simulink model "batu_boost120W_AKIM_KONTROL1"  (R2025a)
settings: Solver=ode23t  StartTime=0.0  StopTime=0.2  RelTol=1e-3
libraries: spsCurrentMeasurementLib x5, spsSeriesRLCBranchLib x3, spsMosfetLib x2, spsVoltageMeasurementLib x2, spsDCVoltageSourceLib x1, spsMeanLib x1, slpidlib x1, spsPWMGeneratorDCDCLib x1, sps_lib x1
settings Model: Creator=sagda  LastModifiedBy=sagda

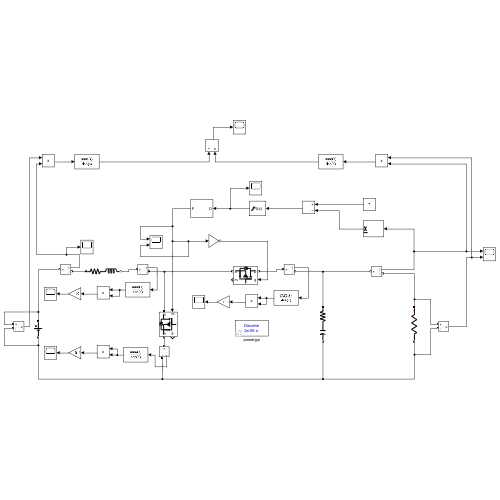
[thumbnail: Simulink's stored preview of the top-level diagram]
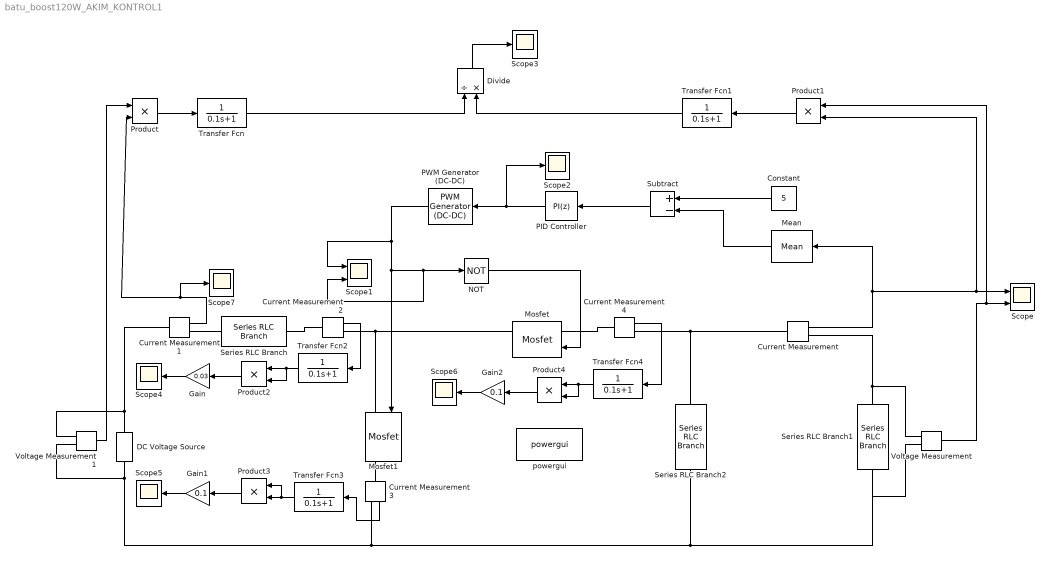
== system batu_boost120W_AKIM_KONTROL1 ==
  Constant : Constant  Value=5
  Current Measurement{,1..4} (5 alike) : spsCurrentMeasurementLib/Current Measurement  PhasorSimulation=off  OutputType=Complex  PSBequivalent=0
  DC Voltage Source : spsDCVoltageSourceLib/DC Voltage Source  Amplitude=24  Measurements=None
  Divide : Product  Inputs=/*
  Gain : Gain  Gain=0.03
  Gain1 : Gain  Gain=0.1
  Gain2 : Gain  Gain=0.1
  Mean : spsMeanLib/Mean  Freq=30000  Vinit=0  Ts=0
  Mosfet : spsMosfetLib/Mosfet  Ron=0.1  Lon=0  Rd=0.01  Vfd=0  IC=0  Rs=1e5  Cs=inf  Measurements=on
  Mosfet1 : spsMosfetLib/Mosfet  Ron=0.1  Lon=0  Rd=0.01  Vfd=0  IC=0  Rs=1e5  Cs=inf  Measurements=on
  NOT : Logic  Operator=NOT  IconShape=distinctive  AllPortsSameDT=off  OutDataTypeStr=boolean
  PID Controller : slpidlib/PID Controller  Controller=PI  Form=Parallel  TimeDomain=Discrete-time  UseExternalTs=off  SampleTime=2e-5  IntegratorMethod=Forward Euler  FilterMethod=Forward Euler  ControllerParametersSource=internal  P=0.001  I=5  UseKiTs=off  D=0  UseExternalDerivativeSource=off  N=100  UseFilter=on  TunerSelectOption=Transfer Function Based (PID Tuner App)  InitialConditionSource=internal  InitialConditionForIntegrator=0  InitialConditionForFilter=0  DifferentiatorICPrevScaledInput=0  ExternalReset=none  TrackingMode=off  Kt=1  LimitOutput=on  SatLimitsSource=internal  UpperSaturationLimit=0.9  LowerSaturationLimit=0  LinearizeAsGain=on  AntiWindupMode=clamping  Kb=1  LimitIntegrator=on  UpperIntegratorSaturationLimit=0.9  LowerIntegratorSaturationLimit=0  POutMin=[]  POutMax=[]  IOutMin=[]  IOutMax=[]  DOutMin=[]  DOutMax=[]  NOutMin=[]  NOutMax=[]  SumOutMin=[]  SumOutMax=[]  SaturationOutMin=[]  SaturationOutMax=[]  PParamMin=[]  PParamMax=[]  IParamMin=[]  IParamMax=[]  DParamMin=[]  DParamMax=[]  NParamMin=[]  NParamMax=[]  KbParamMin=[]  KbParamMax=[]  KtParamMin=[]  KtParamMax=[]  KbOutMin=[]  KbOutMax=[]  KtOutMin=[]  KtOutMax=[]  IntegratorOutMin=[]  IntegratorOutMax=[]  FilterOutMin=[]  FilterOutMax=[]  SumI1OutMin=[]  SumI1OutMax=[]  SumI2OutMin=[]  SumI2OutMax=[]  SumI3OutMin=[]  SumI3OutMax=[]  SumI4OutMin=[]  SumI4OutMax=[]  SumDOutMin=[]  SumDOutMax=[]  DifferentiatorOutMin=[]  DifferentiatorOutMax=[]  FilterDiffOutCoefMin=[]  FilterDiffOutCoefMax=[]  ReciprocalOutMin=[]  ReciprocalOutMax=[]  SumDenOutMin=[]  SumDenOutMax=[]  SumNumOutMin=[]  SumNumOutMax=[]  DivideOutMin=[]  DivideOutMax=[]  UdiffTsProdOutMin=[]  UdiffTsProdOutMax=[]  NTsProdOutMin=[]  NTsProdOutMax=[]  UintegralTsProdOutMin=[]  UintegralTsProdOutMax=[]  UngainTsProdOutMin=[]  UngainTsProdOutMax=[]  ClampingZeroOutDataTypeStr=Inherit: Inherit via back propagation  ClampingZeroOutMin=[]  ClampingZeroOutMax=[]  FilterDenConstantOutDataTypeStr=Inherit: Inherit via back propagation  FilterDenConstantOutMin=[]  FilterDenConstantOutMax=[]  PCopyOutDataTypeStr=Inherit: Inherit via back propagation  PCopyOutMin=[]  PCopyOutMax=[]  NCopyOutDataTypeStr=Inherit: Inherit via back propagation  NCopyOutMin=[]  NCopyOutMax=[]  IntegratorContinuousStateAttributes=''  IntegratorStateMustResolveToSignalObject=off  IntegratorRTWStateStorageClass=Auto  FilterContinuousStateAttributes=''  FilterStateMustResolveToSignalObject=off  FilterRTWStateStorageClass=Auto  ParallelPVariant=InternalParameters  IdealPVariant=Disabled  IVariant=InternalParameters  DVariant=Disabled  IntegratorVariant=Discrete  SatVariant=Enabled  AWVariant=DiscClampingParallel  PCopyVariant=Disabled  TRVariant=Disabled  FdbkBlocksVariant=Forward  IdealPFdbkVariant=Disabled  SatFdbkVariant=Disabled  DerivativeFilterVariant=Disabled  NVariant=Disabled  NCopyVariant=Disabled_SignalSpec  FilterICVariant=Disabled  IntegratorICVariant=InternalICs  ExternalResetVariant=Disabled  TRSumVariant=Passthrough  SumFdbkVariant=Disabled  SumVariant=Sum_PI  TsampFilterVariant=InternalTs  TsampNgainVariant=Passthrough  TsampIntegralVariant=Disabled_SignalSpec  ExternalSaturationOutDataTypeStr=Inherit: Same as second input  DerivativeSourceVariant=Disabled  PreIntVariant=InternalPreInt
  PWM Generator (DC-DC) : spsPWMGeneratorDCDCLib/PWM Generator (DC-DC)  Fsw=5000  Ts=0
  Product{,1..4} (5 alike) : Product
  Scope : Scope  NumInputPorts=2
      settings: ActiveDisplayYMinimum=-127.10682786797719  ActiveDisplayYMaximum=354.81313119342929
  Scope1 : Scope  NumInputPorts=2
      settings: ActiveDisplayYMinimum=0.054276  ActiveDisplayYMaximum=2.1879
  Scope{2..7} (6 alike) : Scope
      Scope2 settings: ActiveDisplayYMinimum=-0.12269  ActiveDisplayYMaximum=1.6409  DataLoggingVariableName=ScopeData2
      Scope3 settings: ActiveDisplayYMinimum=0.94291  ActiveDisplayYMaximum=0.95963  DataLoggingVariableName=ScopeData3
      Scope4 settings: ActiveDisplayYMinimum=0.78588  ActiveDisplayYMaximum=5.2873  DataLoggingVariableName=ScopeData4
      Scope5 settings: ActiveDisplayYMinimum=-0.94871  ActiveDisplayYMaximum=4.3636  DataLoggingVariableName=ScopeData5
      Scope6 settings: ActiveDisplayYMinimum=-13.0591  ActiveDisplayYMaximum=15.0829  DataLoggingVariableName=ScopeData6
      Scope7 settings: ActiveDisplayYMinimum=7.4423  ActiveDisplayYMaximum=25.7483  DataLoggingVariableName=ScopeData7
  Series RLC Branch : spsSeriesRLCBranchLib/Series RLC Branch  LConnTagsString=__new0  RConnTagsString=__new0  BranchType=RL  Resistance=0.03  Inductance=200e-6  SetiL0=off  InitialCurrent=0  Capacitance=1e-6  Setx0=off  InitialVoltage=0  Measurements=None
  Series RLC Branch1 : spsSeriesRLCBranchLib/Series RLC Branch  LConnTagsString=__new0  RConnTagsString=__new0  BranchType=R  Resistance=9.6  Inductance=1e-3  SetiL0=off  InitialCurrent=0  Capacitance=1e-6  Setx0=off  InitialVoltage=0  Measurements=None
  Series RLC Branch2 : spsSeriesRLCBranchLib/Series RLC Branch  LConnTagsString=__new0  RConnTagsString=__new0  BranchType=RC  Resistance=0.02  Inductance=1e-3  SetiL0=off  InitialCurrent=0  Capacitance=220e-6  Setx0=off  InitialVoltage=0  Measurements=None
  Subtract : Sum  Inputs=+-
  Transfer Fcn{,1..4} (5 alike) : TransferFcn  Denominator=[0.1 1]
  Voltage Measurement : spsVoltageMeasurementLib/Voltage Measurement  PhasorSimulation=off  OutputType=Complex  PSBequivalent=0
  Voltage Measurement1 : spsVoltageMeasurementLib/Voltage Measurement  PhasorSimulation=off  OutputType=Complex  PSBequivalent=0
  powergui : sps_lib/powergui  Priority=1  SimulationMode=Discrete  SampleTime=2e-6  frequency=60  Iterations=50  frequencyindice=0  Pbase=100e6  ErrMax=1e-4  UnitsV=kV  UnitsW=MW  buscounter=0  FunctionMessages=off  echomessages=off  EnableUseOfTLC=off  CurrentSourceSwitches=off  DisableSnubberDevices=off  DisableRonSwitches=off  DisableVfSwitches=off  DisplayEquations=off  AutomaticDiscreteSolvers=off  SolverType=Tustin/Backward Euler (TBE)  Interpol=off  ExternalGateDelay=off  methode=off  Ts=100  x0status=blocks  SPID=on  SwTol=0  HookPort=off  NonlinearTolerance=1e-4  nMaxIteration=100  ContinueOnMaxIteration=off  RestoreLinks=warning  ResistiveCurrentMeasurement=off  Frange=[0:2:500]  Ylog=off  Xlog=on  ShowGrid=off  save=off  variable=ZData  structure=0  ZoomFFT=off  StartTime=0.0  cycles=1  DisplayStyle=1  fundamental=60  FreqAxis=off  MaxFrequency=1000  frequencyindicesteady=1  RmsSteady=1  display=off
  wires:
  Voltage Measurement/1 -> Product1/1, Scope/2
  Current Measurement/1 -> Mean/1, Product1/2, Scope/1
  Mean/1 -> Subtract/2
  Constant/1 -> Subtract/1
  Subtract/1 -> PID Controller/1
  PID Controller/1 -> Scope2/1, PWM Generator (DC-DC)/1
  PWM Generator (DC-DC)/1 -> Scope1/1, Mosfet1/1, NOT/1, Scope1/2
  NOT/1 -> Mosfet/1
  Voltage Measurement1/1 -> Product/1
  Current Measurement1/1 -> Scope7/1, Product/2
  Product/1 -> Transfer Fcn/1
  Product1/1 -> Transfer Fcn1/1
  Transfer Fcn/1 -> Divide/1
  Transfer Fcn1/1 -> Divide/2
  Divide/1 -> Scope3/1
  Product2/1 -> Gain/1
  Current Measurement2/1 -> Transfer Fcn2/1
  Gain/1 -> Scope4/1
  Gain1/1 -> Scope5/1
  Current Measurement3/1 -> Transfer Fcn3/1
  Product3/1 -> Gain1/1
  Product4/1 -> Gain2/1
  Current Measurement4/1 -> Transfer Fcn4/1
  Gain2/1 -> Scope6/1
  Transfer Fcn2/1 -> Product2/2, Product2/1
  Transfer Fcn3/1 -> Product3/1, Product3/2
  Transfer Fcn4/1 -> Product4/1, Product4/2
  connections:
  DC Voltage Source/RConn1 -- Current Measurement1/LConn1 -- Voltage Measurement1/LConn1
  Mosfet/RConn1 -- Current Measurement2/RConn1 -- Mosfet1/LConn1
  Voltage Measurement/LConn2 -- Series RLC Branch1/RConn1 -- Series RLC Branch2/RConn1 -- Current Measurement3/RConn1 -- Voltage Measurement1/LConn2 -- DC Voltage Source/LConn1
  Current Measurement4/LConn1 -- Mosfet/LConn1
  Series RLC Branch1/LConn1 -- Voltage Measurement/LConn1 -- Current Measurement/RConn1
  Current Measurement1/RConn1 -- Series RLC Branch/LConn1
  Series RLC Branch/RConn1 -- Current Measurement2/LConn1
  Mosfet1/RConn1 -- Current Measurement3/LConn1
  Current Measurement/LConn1 -- Current Measurement4/RConn1 -- Series RLC Branch2/LConn1
